simulink model "Demo"  (R2019a)
settings: Solver=FixedStepAuto  StartTime=0.0  StopTime=10  RelTol=1e-3
InitFcn:
  | run Initialize.m
StopFcn:
  | run Visualization.m
values from neighbouring files (symbols this model uses):
  K = lqr(A,B,Q,R)    [Initialize.m]
  Ts = 10*10^-3    (= 0.01)    [Initialize.m]
  x0 = [0;    0;  initial_theta_c;  0;   0;  0]    [Initialize.m]
  xr = [1; 0; 0; 0; 0; 0]    [Initialize.m]
settings Model: Creator=visha  LastModifiedBy=visha

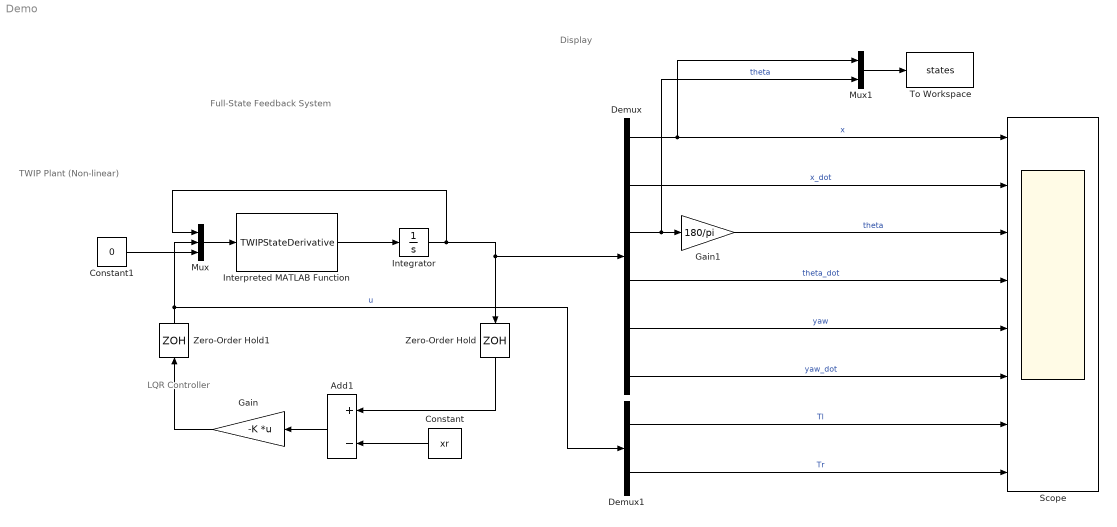
== system Demo ==
  note: Full-State Feedback System
  note: Display
  note: LQR Controller
  note: TWIP Plant (Non-linear)
  Add1 : Sum  Inputs=+-
  Constant : Constant  Value=xr
  Constant1 : Constant  Value=0
  Demux : Demux  Outputs=6
  Demux1 : Demux  Outputs=2
  Gain : Gain  Gain=-K  Multiplication=Matrix(K*u)
  Gain1 : Gain  Gain=180/pi
  Integrator : Integrator  InitialCondition=x0
  Interpreted MATLAB Function : MATLABFcn  MATLABFcn=TWIPStateDerivative
  Mux : Mux  Inputs=3
  Mux1 : Mux  Inputs=2
  Scope : Scope  NumInputPorts=8
  To Workspace : ToWorkspace  VariableName=states  SaveFormat=Timeseries  SampleTime=-1
  Zero-Order Hold : ZeroOrderHold  SampleTime=Ts
  Zero-Order Hold1 : ZeroOrderHold  SampleTime=Ts
  wires:
  Integrator/1 -> Mux/1, Zero-Order Hold/1, Demux/1
  Interpreted MATLAB Function/1 -> Integrator/1
  Add1/1 -> Gain/1
  Constant/1 -> Add1/2
  Mux/1 -> Interpreted MATLAB Function/1
  Demux/4 -> Scope/4  "theta_dot"
  Demux/2 -> Scope/2  "x_dot"
  Demux/1 -> Mux1/1, Scope/1  "x"
  Mux1/1 -> To Workspace/1
  Zero-Order Hold/1 -> Add1/1
  Gain/1 -> Zero-Order Hold1/1
  Zero-Order Hold1/1 -> Demux1/1, Mux/2  "u"
  Gain1/1 -> Scope/3  "theta"
  Demux1/1 -> Scope/7  "Tl"
  Demux1/2 -> Scope/8  "Tr"
  Constant1/1 -> Mux/3
  Demux/6 -> Scope/6  "yaw_dot"
  Demux/5 -> Scope/5  "yaw"
  Demux/3 -> Mux1/2, Gain1/1  "theta"
